simulink model "CHB11"  (R2014b)
settings: Solver=ode45  StartTime=0.0  StopTime=1  RelTol=1e-3
undefined symbols (not defined in the file): freq
libraries: powerlib x22
settings Model: Creator=SELVA  LastModifiedBy=SELVA

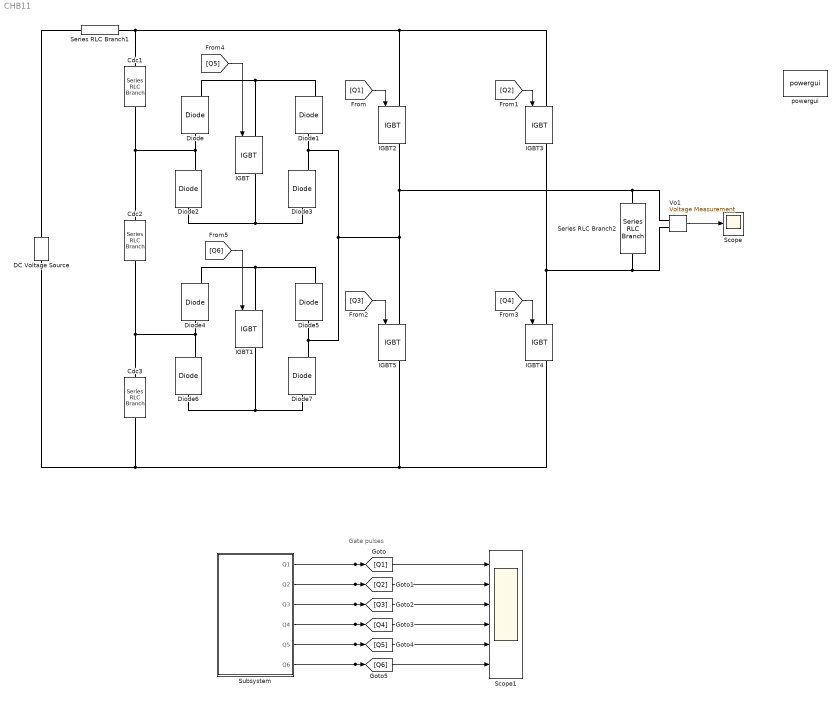
== system CHB11 ==
  note: Gate pulses
  Cdc1 : powerlib/Elements/Series RLC Branch  LConnTagsString=__new0  RConnTagsString=__new0  BranchType=C  Resistance=1  Inductance=1e-3  SetiL0=off  InitialCurrent=0  Capacitance=10e-3  Setx0=off  InitialVoltage=400  Measurements=None
  Cdc2 : powerlib/Elements/Series RLC Branch  LConnTagsString=__new0  RConnTagsString=__new0  BranchType=C  Resistance=1  Inductance=1e-3  SetiL0=off  InitialCurrent=0  Capacitance=10e-3  Setx0=off  InitialVoltage=400  Measurements=None
  Cdc3 : powerlib/Elements/Series RLC Branch  LConnTagsString=__new0  RConnTagsString=__new0  BranchType=C  Resistance=1  Inductance=1e-3  SetiL0=off  InitialCurrent=0  Capacitance=10e-3  Setx0=off  InitialVoltage=400  Measurements=None
  DC Voltage Source : powerlib/Electrical Sources/DC Voltage Source  Amplitude=325.25  Measurements=None
  Diode{,1..7} (8 alike) : powerlib/Power Electronics/Diode  Ron=0.001  Lon=0  Vf=0.8  IC=0  UseSnubber=off  Rs=500  Cs=250e-9  Measurements=on
  IGBT{,1..5} (6 alike) : powerlib/Power Electronics/IGBT  Ron=0.001  Lon=0  Vf=1  Tf=1e-6  Tt=2e-6  IC=0  Rs=1e5  Cs=inf  Measurements=on
  Scope : Scope
      settings: TimeRange=1  YMin=-400  YMax=400  SaveName=ScopeData5
  Scope1 : Scope  NumInputPorts=6
      settings: YMin=0~0~0~0~0~0  YMax=1~1~1~1~1~1  SaveName=ScopeData6
  Series RLC Branch1 : powerlib/Elements/Series RLC Branch  LConnTagsString=__new0  RConnTagsString=__new0  BranchType=R  Resistance=0.001  Inductance=60e-6  SetiL0=off  InitialCurrent=0  Capacitance=0.45e-6  Setx0=off  InitialVoltage=0  Measurements=None
  Series RLC Branch2 : powerlib/Elements/Series RLC Branch  LConnTagsString=__new0  RConnTagsString=__new0  BranchType=R  Resistance=100  Inductance=60e-6  SetiL0=off  InitialCurrent=0  Capacitance=0.45e-6  Setx0=off  InitialVoltage=0  Measurements=None
  Subsystem : Subsystem
  Vo1 : powerlib/Measurements/Voltage Measurement  PhasorSimulation=off  OutputType=Complex  PSBequivalent=0
  powergui : powerlib/powergui  Priority=1  SimulationMode=Continuous  SolverType=Tustin/Backward Euler (TBE)  SampleTime=50e-6  frequency=60  SPID=off  DisableSnubberDevices=off  DisableRonSwitches=off  DisableVfSwitches=off  SwTol=0  DisplayEquations=off  Interpol=off  methode=off  Ts=100  frequencyindice=0  Pbase=100e6  ErrMax=1e-4  Iterations=50  UnitsV=kV  UnitsW=MW  FunctionMessages=off  echomessages=off  HookPort=off  EnableUseOfTLC=off  x0status=blocks  RestoreLinks=warning  ResistiveCurrentMeasurement=off  Frange=[0:2:500]  Ylog=off  Xlog=on  ShowGrid=off  save=off  variable=ZData  structure=0  ZoomFFT=off  StartTime=0.0  cycles=1  DisplayStyle=1  fundamental=60  FreqAxis=off  MaxFrequency=1000  frequencyindicesteady=1  RmsSteady=1  display=off
  wires:
  Subsystem/1(Q1) -> [Q1], Scope1/1
  Subsystem/2(Q2) -> [Q2], Scope1/2
  Subsystem/3(Q3) -> [Q3], Scope1/3
  Subsystem/4(Q4) -> [Q4], Scope1/4
  Subsystem/5(Q5) -> [Q5], Scope1/5
  Subsystem/6(Q6) -> [Q6], Scope1/6
  [Q1] -> IGBT2/1
  [Q2] -> IGBT3/1
  [Q3] -> IGBT5/1
  [Q4] -> IGBT4/1
  [Q5] -> IGBT/1
  [Q6] -> IGBT1/1
  Vo1/1 -> Scope/1
  connections:
  Series RLC Branch1/RConn1 -- Cdc1/LConn1 -- IGBT2/LConn1 -- IGBT3/LConn1
  Diode2/RConn1 -- Diode/LConn1 -- Cdc1/RConn1 -- Cdc2/LConn1
  Diode/RConn1 -- Diode1/RConn1 -- IGBT/LConn1
  IGBT/RConn1 -- Diode3/LConn1 -- Diode2/LConn1
  IGBT1/RConn1 -- Diode7/LConn1 -- Diode6/LConn1
  Diode7/RConn1 -- Diode5/LConn1 -- Diode1/LConn1 -- Diode3/RConn1 -- IGBT5/LConn1 -- Vo1/LConn1 -- Series RLC Branch2/LConn1 -- IGBT2/RConn1
  Diode4/RConn1 -- Diode5/RConn1 -- IGBT1/LConn1
  Diode6/RConn1 -- Diode4/LConn1 -- Cdc2/RConn1 -- Cdc3/LConn1
  IGBT4/RConn1 -- IGBT5/RConn1 -- DC Voltage Source/LConn1 -- Cdc3/RConn1
  Series RLC Branch2/RConn1 -- Vo1/LConn2 -- IGBT4/LConn1 -- IGBT3/RConn1
  Series RLC Branch1/LConn1 -- DC Voltage Source/RConn1

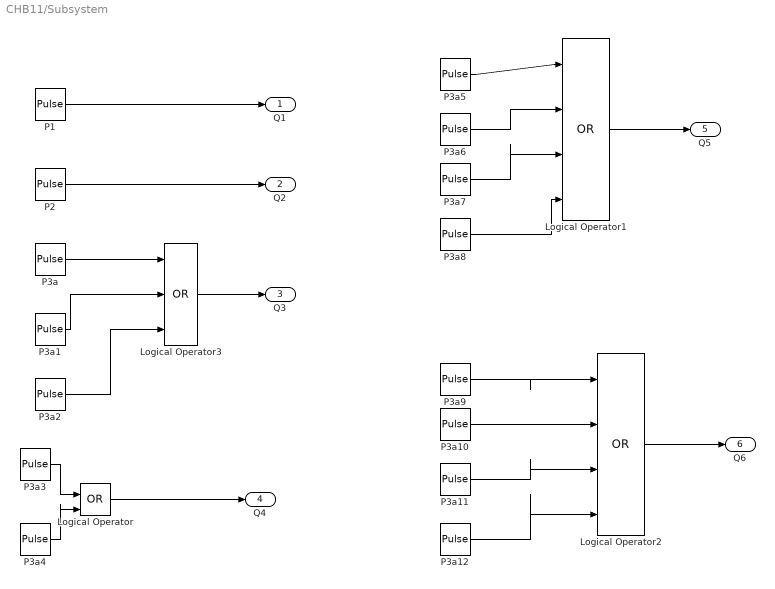
== system CHB11/Subsystem ==
  Logical Operator : Logic  Operator=OR  IconShape=distinctive  AllPortsSameDT=off  OutDataTypeStr=boolean
  Logical Operator1 : Logic  Operator=OR  Inputs=4  IconShape=distinctive  AllPortsSameDT=off  OutDataTypeStr=boolean
  Logical Operator2 : Logic  Operator=OR  Inputs=4  IconShape=distinctive  AllPortsSameDT=off  OutDataTypeStr=boolean
  Logical Operator3 : Logic  Operator=OR  Inputs=3  IconShape=distinctive  AllPortsSameDT=off  OutDataTypeStr=boolean
  P1 : DiscretePulseGenerator  PulseType=Time based  Period=1/freq  PulseWidth=100/12  PhaseDelay=((1/freq)/12)*2
  P2 : DiscretePulseGenerator  PulseType=Time based  Period=1/freq  PulseWidth=(100/12)*5  PhaseDelay=((1/freq)/12)*6
  P3a : DiscretePulseGenerator  PulseType=Time based  Period=1/freq  PulseWidth=100/12  PhaseDelay=((1/freq)/12)*5
  P3a1 : DiscretePulseGenerator  PulseType=Time based  Period=1/freq  PulseWidth=100/12  PhaseDelay=((1/freq)/12)*8
  P3a10 : DiscretePulseGenerator  PulseType=Time based  Period=1/freq  PulseWidth=100/12  PhaseDelay=((1/freq)/12)*4
  P3a11 : DiscretePulseGenerator  PulseType=Time based  Period=1/freq  PulseWidth=100/12  PhaseDelay=((1/freq)/12)*7
  P3a12 : DiscretePulseGenerator  PulseType=Time based  Period=1/freq  PulseWidth=100/12  PhaseDelay=((1/freq)/12)*9
  P3a2 : DiscretePulseGenerator  PulseType=Time based  Period=1/freq  PulseWidth=100/12  PhaseDelay=((1/freq)/12)*11
  P3a3 : DiscretePulseGenerator  PulseType=Time based  Period=1/freq  PulseWidth=(100/12)*6
  P3a4 : DiscretePulseGenerator  PulseType=Time based  Period=1/freq  PulseWidth=100/12  PhaseDelay=((1/freq)/12)*11
  P3a5 : DiscretePulseGenerator  PulseType=Time based  Period=1/freq  PulseWidth=100/12  PhaseDelay=((1/freq)/12)
  P3a6 : DiscretePulseGenerator  PulseType=Time based  Period=1/freq  PulseWidth=100/12  PhaseDelay=((1/freq)/12)*3
  P3a7 : DiscretePulseGenerator  PulseType=Time based  Period=1/freq  PulseWidth=100/12  PhaseDelay=((1/freq)/12)*6
  P3a8 : DiscretePulseGenerator  PulseType=Time based  Period=1/freq  PulseWidth=100/12  PhaseDelay=((1/freq)/12)*10
  P3a9 : DiscretePulseGenerator  PulseType=Time based  Period=1/freq  PulseWidth=100/12
  Q1 : Outport
  Q2 : Outport  Port=2
  Q3 : Outport  Port=3
  Q4 : Outport  Port=4
  Q5 : Outport  Port=5
  Q6 : Outport  Port=6
  wires:
  P1/1 -> Q1/1
  P3a3/1 -> Logical Operator/1
  P3a4/1 -> Logical Operator/2
  Logical Operator/1 -> Q4/1
  Logical Operator2/1 -> Q6/1
  P2/1 -> Q2/1
  Logical Operator1/1 -> Q5/1
  P3a/1 -> Logical Operator3/1
  P3a1/1 -> Logical Operator3/2
  P3a2/1 -> Logical Operator3/3
  Logical Operator3/1 -> Q3/1
  P3a5/1 -> Logical Operator1/1
  P3a6/1 -> Logical Operator1/2
  P3a7/1 -> Logical Operator1/3
  P3a8/1 -> Logical Operator1/4
  P3a9/1 -> Logical Operator2/1
  P3a10/1 -> Logical Operator2/2
  P3a11/1 -> Logical Operator2/3
  P3a12/1 -> Logical Operator2/4
